simulink model "a4_jmavsim_control_smc_wordPic"  (R2023b)
settings: Solver=FixedStepAuto  StartTime=0.0  StopTime=inf  FixedStep=0.01  RelTol=1e-3  EnableMultiTasking=on
undefined symbols (not defined in the file): dev, Main, pwm_output0
libraries: simulink x19, px4uORBlib x3, sharedtransform x1, px4lib x1
settings Model: ExtModeTrigDuration=10  Creator=UAV2  LastModifiedBy=UAV2
settings SolverCC: PositivePriorityOrder=on
settings OptimizationCC: EnhancedBackFolding=on  PassReuseOutputArgsAs=Individual arguments  ZeroExternalMemoryAtStartup=off  ZeroInternalMemoryAtStartup=off  MaxStackSize=64  OptimizeBlockOrder=speed  DifferentSizesBufferReuse=on  EfficientTunableParamExpr=on
settings DebuggingCC: ParameterTunabilityLossMsg=error
settings HardwareCC: ProdBitPerPointer=32  ProdBitPerSizeT=32  ProdBitPerPtrDiffT=32  ProdLargestAtomicInteger=Long  ProdLargestAtomicFloat=Double  ProdWordSize=32  ProdLongLongMode=on  ProdHWDeviceType=ARM Compatible->ARM Cortex
settings SFSimCC: MATLABDynamicMemAlloc=off  SimTargetLang=C++
settings RTWCC: Description=Embedded Coder  SystemTargetFile=ert.tlc  HardwareBoard=PX4 Host Target  TemplateMakefile=ert_default_tmf  Toolchain=GNU Tools for PX4 Autopilots  PortableWordSizes=on  TargetLang=C++
settings CodeAppCC: ForceParamTrailComments=on  IgnoreCustomStorageClasses=off  OperatorAnnotations=on  SimulinkDataObjDesc=on  SFDataObjDesc=on  InsertBlockDesc=on
settings ERTTargetCC: ExtMode=on  ExtModeTransport=2  ExtModeStaticAlloc=on  ExtModeMexFile=ext_xcp  ExtModeMexArgs='127.0.0.1' 1 17725  ExtModeIntrfLevel=Level2 - Open

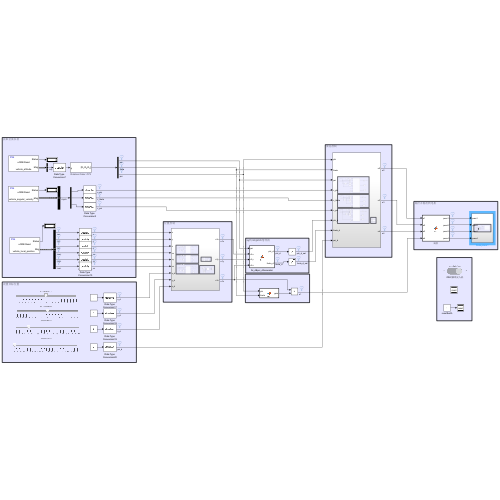
[thumbnail: Simulink's stored preview of the top-level diagram]
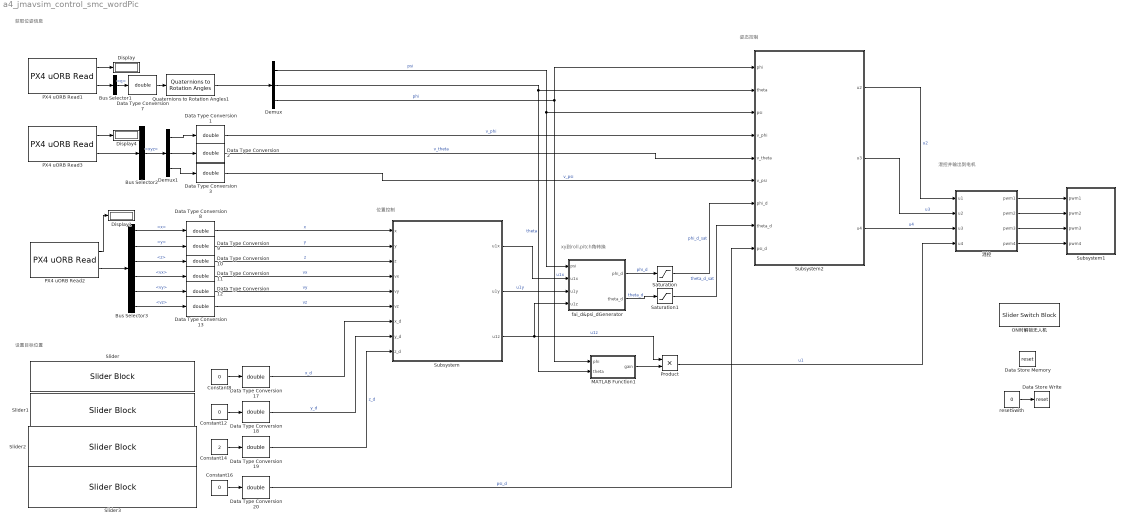
== system a4_jmavsim_control_smc_wordPic ==
  note: 混控并输出到电机
  note: xy到roll,pitch角转换
  note: 姿态控制
  note: 位置控制
  note: 设置目标位置
  note: 获取位姿信息
  Bus Selector1 : BusSelector  OutputSignals=q
  Bus Selector2 : BusSelector  OutputSignals=xyz
  Bus Selector3 : BusSelector  OutputSignals=x,y,z,vx,vy,vz
  Constant12 : Constant  Value=0
  Constant14 : Constant  Value=2
  Constant16 : Constant  Value=0
  Constant8 : Constant  Value=0
  Data Store Memory : DataStoreMemory  DataStoreName=reset  WriteAfterWriteMsg=warning  ShowAdditionalParam=off  OutDataTypeStr=boolean
  Data Store Write : DataStoreWrite  DataStoreName=reset  IndexOptions=Index vector (dialog)  Indices=1  OutputSizes=1
  Data Type Conversion{1..3,7..13,17..20} (14 alike) : DataTypeConversion  OutDataTypeStr=double  SaturateOnIntegerOverflow=off  RndMeth=Floor
  Demux : Demux  Outputs=3
  Demux1 : Demux  Outputs=3
  Display : Display
  Display1 : Display
  Display4 : Display
  MATLAB Function1 : MATLAB Function  TreatAsAtomicUnit=on
  ON时解锁无人机 : SliderSwitchBlock  Description=1时解锁无人机
      settings: Values={{'Off', 'On'}, [1 0]}
  PX4 uORB Read1 : px4uORBlib/PX4 uORB Read  uORBTopic=vehicle_attitude  selectInstance=vehicle_attitude_groundtruth  SampleTime=-1  BlockingMode=off  BlockTimeout=1e-3
  PX4 uORB Read2 : px4uORBlib/PX4 uORB Read  uORBTopic=vehicle_local_position  selectInstance=vehicle_local_position_groundtruth  SampleTime=-1  BlockingMode=off  BlockTimeout=1e-3
  PX4 uORB Read3 : px4uORBlib/PX4 uORB Read  uORBTopic=vehicle_angular_velocity  selectInstance=vehicle_angular_velocity  SampleTime=-1  BlockingMode=off  BlockTimeout=1e-3
  Product : Product
  Quaternions to Rotation Angles1 : sharedtransform/Quaternions to Rotation Angles  rotationOrder=ZYX  aMode=aMode
  Saturation : Saturate
  Saturation1 : Saturate
  Slider : SliderBlock  ScaleMin=-10  ScaleMax=10
  Slider1 : SliderBlock  ScaleMin=-10  ScaleMax=10
  Slider2 : SliderBlock  ScaleMax=10
  Slider3 : SliderBlock  ScaleMax=2
  Subsystem : Subsystem
  Subsystem1 : Subsystem
  Subsystem2 : Subsystem
  fai_d&psi_dGenerator : MATLAB Function  TreatAsAtomicUnit=on
  resetSwith : Constant  Value=0  OutDataTypeStr=boolean
  混控 : MATLAB Function  TreatAsAtomicUnit=on
  wires:
  Quaternions to Rotation Angles1/1 -> Demux/1
  PX4 uORB Read1/1 -> Display/1
  PX4 uORB Read1/2 -> Bus Selector1/1
  Bus Selector1/1 -> Data Type Conversion7/1  "<q>"
  Data Type Conversion7/1 -> Quaternions to Rotation Angles1/1
  resetSwith/1 -> Data Store Write/1
  PX4 uORB Read2/2 -> Bus Selector3/1
  Bus Selector3/2 -> Data Type Conversion9/1  "<y>"
  Bus Selector3/3 -> Data Type Conversion10/1  "<z>"
  Bus Selector3/4 -> Data Type Conversion11/1  "<vx>"
  Bus Selector3/5 -> Data Type Conversion12/1  "<vy>"
  Bus Selector3/6 -> Data Type Conversion13/1  "<vz>"
  Bus Selector3/1 -> Data Type Conversion8/1  "<x>"
  PX4 uORB Read2/1 -> Display1/1
  Subsystem/2(u1y) -> fai_d&psi_dGenerator/3(u1y)  "u1y"
  混控/1(pwm1) -> Subsystem1/1(pwm1)
  混控/2(pwm2) -> Subsystem1/2(pwm2)
  混控/3(pwm3) -> Subsystem1/3(pwm3)
  混控/4(pwm4) -> Subsystem1/4(pwm4)
  Demux/1 -> fai_d&psi_dGenerator/1(psi), Subsystem2/3(psi)  "psi"
  Demux/2 -> MATLAB Function1/2(theta), Subsystem2/2(theta)  "theta"
  Demux/3 -> MATLAB Function1/1(phi), Subsystem2/1(phi)  "phi"
  Constant16/1 -> Data Type Conversion20/1
  Data Type Conversion20/1 -> Subsystem2/9(psi_d)  "psi_d"
  fai_d&psi_dGenerator/1(phi_d) -> Saturation/1  "phi_d"
  fai_d&psi_dGenerator/2(theta_d) -> Saturation1/1  "theta_d"
  Subsystem/3(u1z) -> fai_d&psi_dGenerator/4(u1z), Product/1  "u1z"
  Saturation1/1 -> Subsystem2/8(theta_d)  "theta_d_sat"
  Data Type Conversion8/1 -> Subsystem/1(x)  "x"
  Data Type Conversion9/1 -> Subsystem/2(y)  "y"
  Data Type Conversion10/1 -> Subsystem/3(z)  "z"
  Data Type Conversion12/1 -> Subsystem/5(vy)  "vy"
  Data Type Conversion13/1 -> Subsystem/6(vz)  "vz"
  Data Type Conversion17/1 -> Subsystem/7(x_d)  "x_d"
  Data Type Conversion18/1 -> Subsystem/8(y_d)  "y_d"
  Data Type Conversion19/1 -> Subsystem/9(z_d)  "z_d"
  Data Type Conversion11/1 -> Subsystem/4(vx)  "vx"
  Subsystem/1(u1x) -> fai_d&psi_dGenerator/2(u1x)  "u1x"
  PX4 uORB Read3/2 -> Bus Selector2/1
  PX4 uORB Read3/1 -> Display4/1
  Data Type Conversion1/1 -> Subsystem2/4(v_phi)  "v_phi"
  Data Type Conversion2/1 -> Subsystem2/5(v_theta)  "v_theta"
  Data Type Conversion3/1 -> Subsystem2/6(v_psi)  "v_psi"
  Bus Selector2/1 -> Demux1/1  "<xyz>"
  Demux1/1 -> Data Type Conversion1/1
  Demux1/2 -> Data Type Conversion2/1
  Demux1/3 -> Data Type Conversion3/1
  Saturation/1 -> Subsystem2/7(phi_d)  "phi_d_sat"
  Subsystem2/3(u4) -> 混控/3(u3)  "u4"
  Subsystem2/1(u2) -> 混控/1(u1)  "u2"
  Subsystem2/2(u3) -> 混控/2(u2)  "u3"
  MATLAB Function1/1(gain) -> Product/2
  Product/1 -> 混控/4(u4)  "u1"
  Constant14/1 -> Data Type Conversion19/1
  Constant12/1 -> Data Type Conversion18/1
  Constant8/1 -> Data Type Conversion17/1

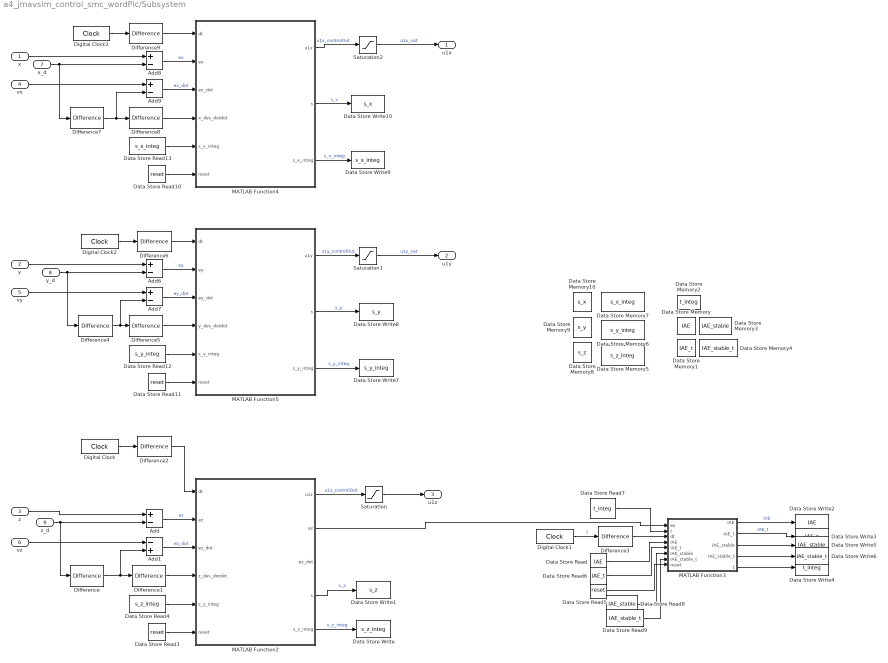
== system a4_jmavsim_control_smc_wordPic/Subsystem ==
  x : Inport
  y : Inport  Port=2
  z : Inport  Port=3
  vx : Inport  Port=4
  vy : Inport  Port=5
  vz : Inport  Port=6
  x_d : Inport  Port=7
  y_d : Inport  Port=8
  z_d : Inport  Port=9
  Add{,6..9} (5 alike) : Sum  Inputs=+-
  Add1 : Sum  Inputs=-+
  Data Store Memory : DataStoreMemory  DataStoreName=IAE  WriteAfterWriteMsg=warning  ShowAdditionalParam=off
  Data Store Memory1 : DataStoreMemory  DataStoreName=IAE_t  WriteAfterWriteMsg=warning  ShowAdditionalParam=off
  Data Store Memory10 : DataStoreMemory  DataStoreName=s_x  WriteAfterWriteMsg=warning  ShowAdditionalParam=off  OutDataTypeStr=double
  Data Store Memory2 : DataStoreMemory  DataStoreName=t_integ  WriteAfterWriteMsg=warning  ShowAdditionalParam=off
  Data Store Memory3 : DataStoreMemory  DataStoreName=IAE_stable  WriteAfterWriteMsg=warning  ShowAdditionalParam=off
  Data Store Memory4 : DataStoreMemory  DataStoreName=IAE_stable_t  WriteAfterWriteMsg=warning  ShowAdditionalParam=off
  Data Store Memory5 : DataStoreMemory  DataStoreName=s_z_integ  WriteAfterWriteMsg=warning  ShowAdditionalParam=off  OutDataTypeStr=double
  Data Store Memory6 : DataStoreMemory  DataStoreName=s_y_integ  WriteAfterWriteMsg=warning  ShowAdditionalParam=off  OutDataTypeStr=double
  Data Store Memory7 : DataStoreMemory  DataStoreName=s_x_integ  WriteAfterWriteMsg=warning  ShowAdditionalParam=off  OutDataTypeStr=double
  Data Store Memory8 : DataStoreMemory  DataStoreName=s_z  WriteAfterWriteMsg=warning  ShowAdditionalParam=off  OutDataTypeStr=double
  Data Store Memory9 : DataStoreMemory  DataStoreName=s_y  WriteAfterWriteMsg=warning  ShowAdditionalParam=off  OutDataTypeStr=double
  Data Store Read : DataStoreRead  DataStoreName=IAE  IndexOptions=Index vector (dialog)  Indices=1  OutputSizes=1
  Data Store Read{3,5,10..11} (4 alike) : DataStoreRead  DataStoreName=reset  IndexOptions=Index vector (dialog)  Indices=1  OutputSizes=1
  Data Store Read12 : DataStoreRead  DataStoreName=s_y_integ  IndexOptions=Index vector (dialog)  Indices=1  OutputSizes=1
  Data Store Read13 : DataStoreRead  DataStoreName=s_x_integ  IndexOptions=Index vector (dialog)  Indices=1  OutputSizes=1
  Data Store Read4 : DataStoreRead  DataStoreName=s_z_integ  IndexOptions=Index vector (dialog)  Indices=1  OutputSizes=1
  Data Store Read6 : DataStoreRead  DataStoreName=IAE_t  IndexOptions=Index vector (dialog)  Indices=1  OutputSizes=1
  Data Store Read7 : DataStoreRead  DataStoreName=t_integ  IndexOptions=Index vector (dialog)  Indices=1  OutputSizes=1
  Data Store Read8 : DataStoreRead  DataStoreName=IAE_stable  IndexOptions=Index vector (dialog)  Indices=1  OutputSizes=1
  Data Store Read9 : DataStoreRead  DataStoreName=IAE_stable_t  IndexOptions=Index vector (dialog)  Indices=1  OutputSizes=1
  Data Store Write : DataStoreWrite  DataStoreName=s_z_integ  IndexOptions=Index vector (dialog)  Indices=1  OutputSizes=1
  Data Store Write1 : DataStoreWrite  DataStoreName=s_z  IndexOptions=Index vector (dialog)  Indices=1  OutputSizes=1
  Data Store Write10 : DataStoreWrite  DataStoreName=s_x  IndexOptions=Index vector (dialog)  Indices=1  OutputSizes=1
  Data Store Write2 : DataStoreWrite  DataStoreName=IAE  IndexOptions=Index vector (dialog)  Indices=1  OutputSizes=1
  Data Store Write3 : DataStoreWrite  DataStoreName=IAE_t  IndexOptions=Index vector (dialog)  Indices=1  OutputSizes=1
  Data Store Write4 : DataStoreWrite  DataStoreName=t_integ  IndexOptions=Index vector (dialog)  Indices=1  OutputSizes=1
  Data Store Write5 : DataStoreWrite  DataStoreName=IAE_stable  IndexOptions=Index vector (dialog)  Indices=1  OutputSizes=1
  Data Store Write6 : DataStoreWrite  DataStoreName=IAE_stable_t  IndexOptions=Index vector (dialog)  Indices=1  OutputSizes=1
  Data Store Write7 : DataStoreWrite  DataStoreName=s_y_integ  IndexOptions=Index vector (dialog)  Indices=1  OutputSizes=1
  Data Store Write8 : DataStoreWrite  DataStoreName=s_y  IndexOptions=Index vector (dialog)  Indices=1  OutputSizes=1
  Data Store Write9 : DataStoreWrite  DataStoreName=s_x_integ  IndexOptions=Index vector (dialog)  Indices=1  OutputSizes=1
  Difference{,1..9} (10 alike) : simulink/Discrete/Difference  ICPrevInput=0.0  OutMin=[]  OutMax=[]  OutDataType=fixdt(1, 16)  OutScaling=2^-10  DoSatur=off
  Digital Clock{,1..3} (4 alike) : DigitalClock  SampleTime=0.01
  MATLAB Function2 : MATLAB Function  TreatAsAtomicUnit=on
  MATLAB Function3 : MATLAB Function  TreatAsAtomicUnit=on
  MATLAB Function4 : MATLAB Function  TreatAsAtomicUnit=on
  MATLAB Function5 : MATLAB Function  TreatAsAtomicUnit=on
  Saturation : Saturate  UpperLimit=1  LowerLimit=0
  Saturation1 : Saturate
  Saturation2 : Saturate  UpperLimit=1  LowerLimit=-1
  u1x : Outport
  u1y : Outport  Port=2
  u1z : Outport  Port=3
  wires:
  MATLAB Function2/1(u1z) -> Saturation/1  "u1z_controlOut"
  Difference/1 -> Add1/2, Difference1/1
  Difference1/1 -> MATLAB Function2/4(z_des_dotdot)
  Data Store Read3/1 -> MATLAB Function2/6(reset)
  Data Store Read4/1 -> MATLAB Function2/5("s_z_integ ")
  Digital Clock/1 -> Difference2/1
  Difference2/1 -> MATLAB Function2/1(dt)
  MATLAB Function2/4(s) -> Data Store Write1/1  "s_z"
  MATLAB Function2/5(s_z_integ) -> Data Store Write/1  "s_z_integ"
  MATLAB Function2/2(ez) -> MATLAB Function3/1(ez)
  Saturation/1 -> u1z/1
  Add/1 -> MATLAB Function2/2("ez ")  "ez"
  z_d/1 -> Add/2, Difference/1
  vz/1 -> Add1/1
  Add1/1 -> MATLAB Function2/3("ez_dot ")  "ez_dot"
  Data Store Read5/1 -> MATLAB Function3/8(reset)
  Difference3/1 -> MATLAB Function3/3(dt)
  MATLAB Function3/1(IAE) -> Data Store Write2/1  "IAE"
  MATLAB Function3/2(IAE_t) -> Data Store Write3/1  "IAE_t"
  Digital Clock1/1 -> Difference3/1  "t"
  Data Store Read/1 -> MATLAB Function3/4("IAE ")
  Data Store Read6/1 -> MATLAB Function3/5("IAE_t ")
  Data Store Read7/1 -> MATLAB Function3/2("t ")
  MATLAB Function3/5(t) -> Data Store Write4/1
  MATLAB Function3/3(IAE_stable) -> Data Store Write5/1
  MATLAB Function3/4(IAE_stable_t) -> Data Store Write6/1
  Data Store Read8/1 -> MATLAB Function3/6("IAE_stable ")
  Data Store Read9/1 -> MATLAB Function3/7("IAE_stable_t ")
  Add7/1 -> MATLAB Function5/3(ey_dot)  "ey_dot"
  Difference4/1 -> Add7/2, Difference5/1
  Data Store Read12/1 -> MATLAB Function5/5("s_y_integ ")
  MATLAB Function5/1(u1y) -> Saturation1/1  "u1y_controlOut"
  Data Store Read11/1 -> MATLAB Function5/6(reset)
  MATLAB Function5/3(s_y_integ) -> Data Store Write7/1  "s_y_integ"
  Difference5/1 -> MATLAB Function5/4(y_des_dotdot)
  Digital Clock2/1 -> Difference6/1
  vy/1 -> Add7/1
  Add6/1 -> MATLAB Function5/2(ey)  "ey"
  Saturation1/1 -> u1y/1  "u1y_sat"
  Difference6/1 -> MATLAB Function5/1(dt)
  y/1 -> Add6/1
  MATLAB Function5/2(s) -> Data Store Write8/1  "s_y"
  Difference8/1 -> MATLAB Function4/4(x_des_dotdot)
  Data Store Read10/1 -> MATLAB Function4/6(reset)
  MATLAB Function4/1(u1x) -> Saturation2/1  "u1x_controlOut"
  Data Store Read13/1 -> MATLAB Function4/5("s_x_integ ")
  Difference7/1 -> Add9/2, Difference8/1
  Add9/1 -> MATLAB Function4/3(ex_dot)  "ex_dot"
  Saturation2/1 -> u1x/1  "u1x_sat"
  MATLAB Function4/3(s_x_integ) -> Data Store Write9/1  "s_x_integ"
  Digital Clock3/1 -> Difference9/1
  Add8/1 -> MATLAB Function4/2(ex)  "ex"
  Difference9/1 -> MATLAB Function4/1(dt)
  MATLAB Function4/2(s) -> Data Store Write10/1  "s_x"
  z/1 -> Add/1
  x/1 -> Add8/1
  vx/1 -> Add9/1
  x_d/1 -> Add8/2, Difference7/1
  y_d/1 -> Add6/2, Difference4/1

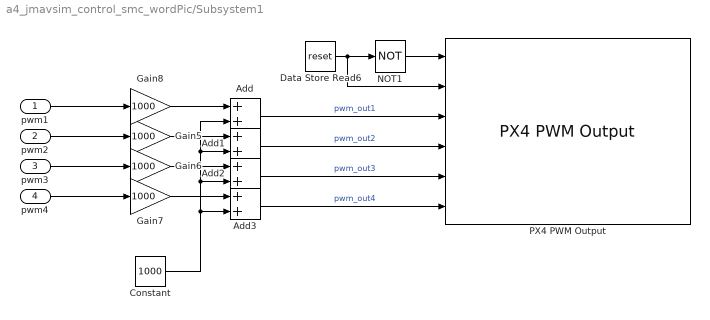
== system a4_jmavsim_control_smc_wordPic/Subsystem1 ==
  pwm1 : Inport
  pwm2 : Inport  Port=2
  pwm3 : Inport  Port=3
  pwm4 : Inport  Port=4
  Add{,1..3} (4 alike) : Sum  OutDataTypeStr=uint16
  Constant : Constant  Value=1000
  Data Store Read6 : DataStoreRead  DataStoreName=reset  IndexOptions=Index vector (dialog)  Indices=1  OutputSizes=1
  Gain{5..8} (4 alike) : Gain  Gain=1000  OutDataTypeStr=uint16
  NOT1 : Logic  Operator=NOT  IconShape=distinctive  AllPortsSameDT=off  OutDataTypeStr=boolean
  PX4 PWM Output : px4lib/PX4 PWM Output  pwmDevice=Main (/dev/pwm_output0)  pwmChannel1_=on  pwmChannel2_=on  pwmChannel3_=on  pwmChannel4_=on  pwmChannel5_=off  pwmChannel6_=off  pwmChannel7_=off  pwmChannel8_=off  forceTerminateFailsafe=off  outputErrorStatus=off
  wires:
  NOT1/1 -> PX4 PWM Output/1
  Add3/1 -> PX4 PWM Output/6  "pwm_out4"
  Data Store Read6/1 -> PX4 PWM Output/2, NOT1/1
  Add/1 -> PX4 PWM Output/3  "pwm_out1"
  Add1/1 -> PX4 PWM Output/4  "pwm_out2"
  pwm3/1 -> Gain6/1
  pwm1/1 -> Gain8/1
  pwm2/1 -> Gain5/1
  pwm4/1 -> Gain7/1
  Add2/1 -> PX4 PWM Output/5  "pwm_out3"
  Gain8/1 -> Add/1
  Constant/1 -> Add3/2, Add2/2, Add1/2, Add/2
  Gain5/1 -> Add1/1
  Gain7/1 -> Add3/1
  Gain6/1 -> Add2/1

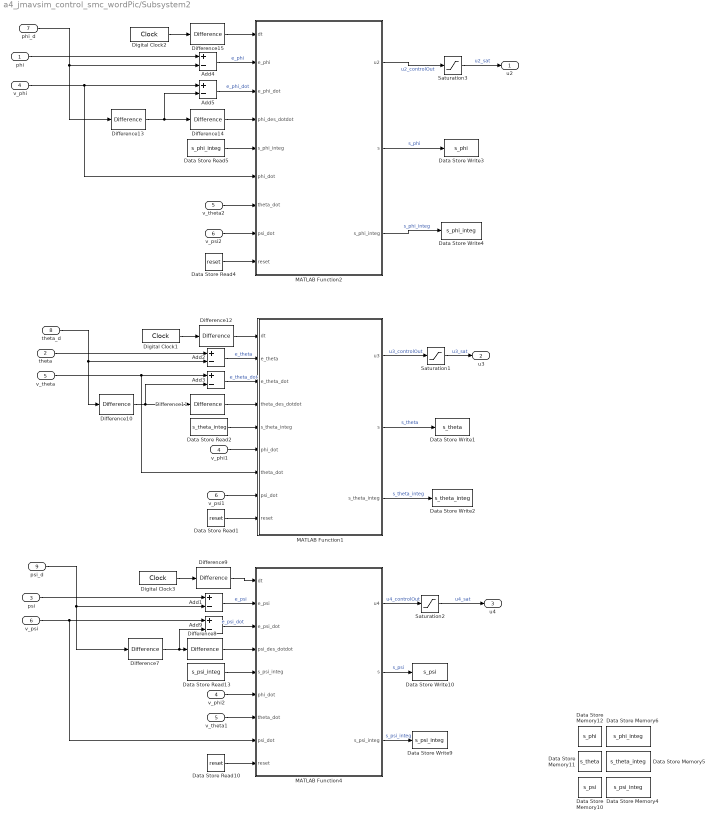
== system a4_jmavsim_control_smc_wordPic/Subsystem2 ==
  phi : Inport
  theta : Inport  Port=2
  psi : Inport  Port=3
  v_phi : Inport  Port=4
  v_theta : Inport  Port=5
  v_psi : Inport  Port=6
  phi_d : Inport  Port=7
  theta_d : Inport  Port=8
  psi_d : Inport  Port=9
  Add{1..5,9} (6 alike) : Sum  Inputs=+-
  Data Store Memory10 : DataStoreMemory  DataStoreName=s_psi  WriteAfterWriteMsg=warning  ShowAdditionalParam=off  OutDataTypeStr=double
  Data Store Memory11 : DataStoreMemory  DataStoreName=s_theta  WriteAfterWriteMsg=warning  ShowAdditionalParam=off  OutDataTypeStr=double
  Data Store Memory12 : DataStoreMemory  DataStoreName=s_phi  WriteAfterWriteMsg=warning  ShowAdditionalParam=off  OutDataTypeStr=double
  Data Store Memory4 : DataStoreMemory  DataStoreName=s_psi_integ  WriteAfterWriteMsg=warning  ShowAdditionalParam=off  OutDataTypeStr=double
  Data Store Memory5 : DataStoreMemory  DataStoreName=s_theta_integ  WriteAfterWriteMsg=warning  ShowAdditionalParam=off  OutDataTypeStr=double
  Data Store Memory6 : DataStoreMemory  DataStoreName=s_phi_integ  WriteAfterWriteMsg=warning  ShowAdditionalParam=off  OutDataTypeStr=double
  Data Store Read1 : DataStoreRead  DataStoreName=reset  IndexOptions=Index vector (dialog)  Indices=1  OutputSizes=1
  Data Store Read10 : DataStoreRead  DataStoreName=reset  IndexOptions=Index vector (dialog)  Indices=1  OutputSizes=1
  Data Store Read13 : DataStoreRead  DataStoreName=s_psi_integ  IndexOptions=Index vector (dialog)  Indices=1  OutputSizes=1
  Data Store Read2 : DataStoreRead  DataStoreName=s_theta_integ  IndexOptions=Index vector (dialog)  Indices=1  OutputSizes=1
  Data Store Read4 : DataStoreRead  DataStoreName=reset  IndexOptions=Index vector (dialog)  Indices=1  OutputSizes=1
  Data Store Read5 : DataStoreRead  DataStoreName=s_phi_integ  IndexOptions=Index vector (dialog)  Indices=1  OutputSizes=1
  Data Store Write1 : DataStoreWrite  DataStoreName=s_theta  IndexOptions=Index vector (dialog)  Indices=1  OutputSizes=1
  Data Store Write10 : DataStoreWrite  DataStoreName=s_psi  IndexOptions=Index vector (dialog)  Indices=1  OutputSizes=1
  Data Store Write2 : DataStoreWrite  DataStoreName=s_theta_integ  IndexOptions=Index vector (dialog)  Indices=1  OutputSizes=1
  Data Store Write3 : DataStoreWrite  DataStoreName=s_phi  IndexOptions=Index vector (dialog)  Indices=1  OutputSizes=1
  Data Store Write4 : DataStoreWrite  DataStoreName=s_phi_integ  IndexOptions=Index vector (dialog)  Indices=1  OutputSizes=1
  Data Store Write9 : DataStoreWrite  DataStoreName=s_psi_integ  IndexOptions=Index vector (dialog)  Indices=1  OutputSizes=1
  Difference{7..15} (9 alike) : simulink/Discrete/Difference  ICPrevInput=0.0  OutMin=[]  OutMax=[]  OutDataType=fixdt(1, 16)  OutScaling=2^-10  DoSatur=off
  Digital Clock1 : DigitalClock  SampleTime=0.01
  Digital Clock2 : DigitalClock  SampleTime=0.01
  Digital Clock3 : DigitalClock  SampleTime=0.01
  MATLAB Function1 : MATLAB Function  TreatAsAtomicUnit=on
  MATLAB Function2 : MATLAB Function  TreatAsAtomicUnit=on
  MATLAB Function4 : MATLAB Function  TreatAsAtomicUnit=on
  Saturation1 : Saturate  UpperLimit=0.1  LowerLimit=-0.1
  Saturation2 : Saturate  UpperLimit=0.2  LowerLimit=-0.2
  Saturation3 : Saturate  UpperLimit=0.1  LowerLimit=-0.1
  v_phi1 : InportShadow  Port=4
  v_phi2 : InportShadow  Port=4
  v_psi1 : InportShadow  Port=6
  v_psi2 : InportShadow  Port=6
  v_theta1 : InportShadow  Port=5
  v_theta2 : InportShadow  Port=5
  u2 : Outport
  u3 : Outport  Port=2
  u4 : Outport  Port=3
  wires:
  Data Store Read10/1 -> MATLAB Function4/9(reset)
  Data Store Read13/1 -> MATLAB Function4/5("s_psi_integ ")
  MATLAB Function4/3(s_psi_integ) -> Data Store Write9/1  "s_psi_integ"
  Saturation2/1 -> u4/1  "u4_sat"
  Add9/1 -> MATLAB Function4/3(e_psi_dot)  "e_psi_dot"
  Difference7/1 -> Add9/2, Difference8/1
  Difference8/1 -> MATLAB Function4/4(psi_des_dotdot)
  Difference9/1 -> MATLAB Function4/1(dt)
  MATLAB Function4/2(s) -> Data Store Write10/1  "s_psi"
  MATLAB Function4/1(u4) -> Saturation2/1  "u4_controlOut"
  Digital Clock3/1 -> Difference9/1
  psi/1 -> Add1/1
  Add1/1 -> MATLAB Function4/2(e_psi)  "e_psi"
  Difference12/1 -> MATLAB Function1/1(dt)
  Digital Clock1/1 -> Difference12/1
  Difference11/1 -> MATLAB Function1/4(theta_des_dotdot)
  MATLAB Function1/1(u3) -> Saturation1/1  "u3_controlOut"
  Data Store Read2/1 -> MATLAB Function1/5("s_theta_integ ")
  MATLAB Function1/2(s) -> Data Store Write1/1  "s_theta"
  Difference10/1 -> Add3/2, Difference11/1
  Data Store Read1/1 -> MATLAB Function1/9(reset)
  Add2/1 -> MATLAB Function1/2(e_theta)  "e_theta"
  Add3/1 -> MATLAB Function1/3(e_theta_dot)  "e_theta_dot"
  MATLAB Function1/3(s_theta_integ) -> Data Store Write2/1  "s_theta_integ"
  theta/1 -> Add2/1
  Saturation3/1 -> u2/1  "u2_sat"
  phi/1 -> Add4/1
  Difference13/1 -> Add5/2, Difference14/1
  Data Store Read4/1 -> MATLAB Function2/9(reset)
  MATLAB Function2/1(u2) -> Saturation3/1  "u2_controlOut"
  Data Store Read5/1 -> MATLAB Function2/5("s_phi_integ ")
  Difference14/1 -> MATLAB Function2/4(phi_des_dotdot)
  Digital Clock2/1 -> Difference15/1
  Difference15/1 -> MATLAB Function2/1(dt)
  Add5/1 -> MATLAB Function2/3(e_phi_dot)  "e_phi_dot"
  MATLAB Function2/2(s) -> Data Store Write3/1  "s_phi"
  Add4/1 -> MATLAB Function2/2(e_phi)  "e_phi"
  MATLAB Function2/3(s_phi_integ) -> Data Store Write4/1  "s_phi_integ"
  v_phi/1 -> MATLAB Function2/6(phi_dot), Add5/1
  v_theta/1 -> Add3/1, MATLAB Function1/7(theta_dot)
  v_psi/1 -> Add9/1, MATLAB Function4/8(psi_dot)
  v_phi1/1 -> MATLAB Function1/6(phi_dot)
  v_theta2/1 -> MATLAB Function2/7(theta_dot)
  v_psi2/1 -> MATLAB Function2/8(psi_dot)
  v_psi1/1 -> MATLAB Function1/8(psi_dot)
  v_phi2/1 -> MATLAB Function4/6(phi_dot)
  v_theta1/1 -> MATLAB Function4/7(theta_dot)
  Saturation1/1 -> u3/1  "u3_sat"
  psi_d/1 -> Difference7/1, Add1/2
  theta_d/1 -> Difference10/1, Add2/2
  phi_d/1 -> Difference13/1, Add4/2

== matlab function a4_jmavsim_control_smc_wordPic/Subsystem/MATLAB Function5 ==
  data: dt input; ey input double; u1y output double; ey_dot input double; y_des_dotdot input; s_y_integ input; reset input; s output; s_y_integ output
function [u1y, s, s_y_integ] = u1yfcn(dt, ey, ey_dot, y_des_dotdot,...
                    s_y_integ, reset)

if (reset == 1); s_y_integ = 0; end
m = 0.8; g = 9.80665; %Ix = 0.005; Iy = 0.005; Iz = 0.009; L = 0.33 / 2;
Ky = 0;

alpha = 2;beta = 1;gamma = 0.4;
mu = 0.9;r = 5/3;
K=0.1;K1 = 0.5;K2 = 0.5;

s = alpha * ey +  (beta * sign(ey_dot) * (abs(ey_dot)) ^ mu) + (gamma * sign(ey) * (abs(ey)) ^ r);
s_y_integ = s_y_integ + K2 * sign(s) * dt;

u1y = -m*(- Ky/m*ey_dot - y_des_dotdot + alpha/(beta*mu)*sign(ey_dot) * (abs(ey_dot))^(2-mu)...
    + gamma*r/(beta*mu)*(sign(ey) * (abs(ey))^(r-1))* sign(ey_dot) * (abs(ey_dot))^(2-mu) + K1*(abs(s))^(1/2)*sign(s)...
    + s_y_integ);

u1y = u1y * K;

== matlab function a4_jmavsim_control_smc_wordPic/Subsystem2/MATLAB Function4 ==
  data: dt input; e_psi input double; u4 output double; e_psi_dot input double; psi_des_dotdot input; s_psi_integ input; phi_dot input; theta_dot input; psi_dot input; reset input; s output; s_psi_integ output
function [u4, s, s_psi_integ] = u4fcn(dt, e_psi, e_psi_dot, psi_des_dotdot,...
                    s_psi_integ, phi_dot, theta_dot, psi_dot, reset)

if (reset == 1); s_psi_integ = 0; end
m = 0.8; g = 9.80665; Ix = 0.005; Iy = 0.005; Iz = 0.009; L = 0.33 / 2;
Kpsi = 0;

alpha = 2;beta = 1;gamma = 0.4;
mu = 15/17;r = 1.1;
K = 5; K1 = 2; K2 = 2;

s = alpha * e_psi +  real(beta * sign(e_psi_dot) * (abs(e_psi_dot)) ^ mu) + real(gamma * sign(e_psi) * (abs(e_psi)) ^ r);
s_psi_integ = s_psi_integ + K2 * sign(s) * dt;

u4 = -Iz*((Ix-Iy)/Iz*phi_dot*theta_dot - Kpsi/Iz*psi_dot - psi_des_dotdot + alpha/(beta*mu)*sign(e_psi_dot) * (abs(e_psi_dot))^(2-mu)...
    + gamma*r/(beta*mu)*(sign(e_psi) * (abs(e_psi))^(r-1))* sign(e_psi_dot) * (abs(e_psi_dot))^(2-mu) + K1*(abs(s))^(1/2)*sign(s)...
    + s_psi_integ);
u4 = u4 * K;

== matlab function a4_jmavsim_control_smc_wordPic/fai_d&psi_dGenerator ==
  data: psi input double; phi_d output double; u1x input double; u1y input double; u1z input double; theta_d output double
function [phi_d, theta_d] = fcn(psi, u1x, u1y, u1z)

% fai_d = atan((y_d - y)/(x_d - x));
% theta_d = atan((z_d - z)/(((x_d - x)^2 + (y_d - y)^2)^(1/2)));
phi_d = -1 * atan((u1x * sin(psi) - u1y * cos(psi)) / u1z );
theta_d = -1 * atan((u1x * cos(psi) + u1y * sin(psi)) * cos(phi_d) / u1z );

== matlab function a4_jmavsim_control_smc_wordPic/MATLAB Function1 ==
  data: phi input double; gain output double; theta input double
function gain = fcn(phi, theta)

gain = 1/(cos(phi) * cos(theta));

== matlab function a4_jmavsim_control_smc_wordPic/Subsystem2/MATLAB Function1 ==
  data: dt input; e_theta input double; u3 output double; e_theta_dot input double; theta_des_dotdot input; s_theta_integ input; phi_dot input; theta_dot input; psi_dot input; reset input; s output; s_theta_integ output
function [u3, s, s_theta_integ] = u3fcn(dt, e_theta, e_theta_dot, theta_des_dotdot,...
                    s_theta_integ, phi_dot, theta_dot, psi_dot, reset)

if (reset == 1); s_theta_integ = 0; end
m = 0.8; g = 9.80665; Ix = 0.005; Iy = 0.005; Iz = 0.009; L = 0.33 / 2;
Ktheta = 0;

alpha = 2;beta = 1;gamma = 0.4;
mu = 15/17;r = 1.1;
K1 = 5; K2 = (K1^2)/2;

s = alpha * e_theta +  (beta * sign(e_theta_dot) * (abs(e_theta_dot)) ^ mu) + (gamma * sign(e_theta) * (abs(e_theta)) ^ r);
s_theta_integ = s_theta_integ + K2 * sign(s) * dt;

u3 = -Iy*((Iz-Ix)/Iy*phi_dot*psi_dot - Ktheta/Iy*theta_dot - theta_des_dotdot + alpha/(beta*mu)*sign(e_theta_dot) * (abs(e_theta_dot))^(2-mu)...
    + gamma*r/(beta*mu)*(sign(e_theta) * (abs(e_theta))^(r-1))* sign(e_theta_dot) * (abs(e_theta_dot))^(2-mu) + K1*(abs(s))^(1/2)*sign(s)...
    + s_theta_integ);

== matlab function a4_jmavsim_control_smc_wordPic/Subsystem2/MATLAB Function2 ==
  data: dt input; e_phi input double; u2 output double; e_phi_dot input double; phi_des_dotdot input; s_phi_integ input; phi_dot input; theta_dot input; psi_dot input; reset input; s output; s_phi_integ output
function [u2, s, s_phi_integ] = u2fcn(dt, e_phi, e_phi_dot, phi_des_dotdot,...
                    s_phi_integ, phi_dot, theta_dot, psi_dot, reset)

if (reset == 1); s_phi_integ = 0; end
m = 0.8; g = 9.80665; Ix = 0.005; Iy = 0.005; Iz = 0.009; L = 0.33 / 2;
Kphi = 0;

alpha = 2;beta = 1;gamma = 0.4;
mu = 15/17;r = 1.1;
K1 = 5; K2 = (K1^2)/2;

s = alpha * e_phi +  (beta * sign(e_phi_dot) * (abs(e_phi_dot)) ^ mu) + (gamma * sign(e_phi) * (abs(e_phi)) ^ r);
s_phi_integ = s_phi_integ + K2 * sign(s) * dt;

u2 = -Ix*((Iy-Iz)/Ix*theta_dot*psi_dot - Kphi/Ix*phi_dot - phi_des_dotdot + alpha/(beta*mu)*sign(e_phi_dot) * (abs(e_phi_dot))^(2-mu)...
    + gamma*r/(beta*mu)*(sign(e_phi) * (abs(e_phi))^(r-1))* sign(e_phi_dot) * (abs(e_phi_dot))^(2-mu) + K1*(abs(s))^(1/2)*sign(s)...
    + s_phi_integ);

== matlab function a4_jmavsim_control_smc_wordPic/混控 ==
  data: u1 input double; pwm1 output double; u2 input double; u3 input double; u4 input double; pwm2 output double; pwm3 output; pwm4 output
function [pwm1,pwm2,pwm3,pwm4] = fcn(u1, u2, u3, u4)

convertMatrix = [-1/sqrt(2)     1/sqrt(2)   1 1;
                1/sqrt(2)       -1/sqrt(2)  1 1;
                1/sqrt(2)       1/sqrt(2)  -1 1;
                -1/sqrt(2)      -1/sqrt(2) -1 1];
pwm = convertMatrix * [u1; u2; u3; u4];
pwm1 = pwm(1);
pwm2 = pwm(2);
pwm3 = pwm(3);
pwm4 = pwm(4);

== matlab function a4_jmavsim_control_smc_wordPic/Subsystem/MATLAB Function2 ==
  data: dt input; ez input double; u1z output double; ez output; ez_dot output; ez_dot input double; z_des_dotdot input; s_z_integ input; reset input; s output; s_z_integ output
function [u1z, ez, ez_dot, s, s_z_integ] = u1zfcn(dt, ez, ez_dot, z_des_dotdot,...
                    s_z_integ, reset)

if (reset == 1); s_z_integ = 0; end
m = 0.8; g = 9.80665; %Ix = 0.005; Iy = 0.005; Iz = 0.009; L = 0.33 / 2;
Kz = 0;

alpha = 2;beta = 1;gamma = 0.4;
mu = 0.9;r = 5/3;
K=2;K1 = 1;K2 = 1;

s = alpha * ez +  (beta * sign(ez_dot) * (abs(ez_dot)) ^ mu) + (gamma * sign(ez) * (abs(ez)) ^ r);
s_z_integ = s_z_integ + K2 * sign(s) * dt;

u1z = -m*(-g - Kz/m*ez_dot - z_des_dotdot + alpha/(beta*mu)*sign(ez_dot) * (abs(ez_dot))^(2-mu)...
    + gamma*r/(beta*mu)*(sign(ez) * (abs(ez))^(r-1))* sign(ez_dot) * (abs(ez_dot))^(2-mu) + K1*(abs(s))^(1/2)*sign(s)...
    + s_z_integ);

u1z = u1z/(K*m*g);

== matlab function a4_jmavsim_control_smc_wordPic/Subsystem/MATLAB Function3 ==
  data: ez input double; t input; IAE output; dt input double; IAE input; IAE_t input; IAE_stable input; IAE_stable_t input; reset input; IAE_t output; IAE_stable output; IAE_stable_t output; t output
function [IAE, IAE_t, IAE_stable, IAE_stable_t, t]  = fcn(ez, t, dt, IAE, IAE_t, IAE_stable, IAE_stable_t, reset)

if (reset == 1); t = 0; IAE = 0; IAE_stable = 0; IAE_t = 0; IAE_stable_t = 0; end

t = t + dt;
if (t < 5.01); IAE = IAE + sqrt(ez^2)*dt; end

if (t > 5.00 && t < 10.01); IAE_stable = IAE_stable + sqrt(ez^2)*dt; end

if (t > 4.99 && t < 5.01); IAE_t =  IAE / t; end

if (t > 9.99 && t < 10.01); IAE_stable_t =  IAE_stable / 5; end

== matlab function a4_jmavsim_control_smc_wordPic/Subsystem/MATLAB Function4 ==
  data: dt input; ex input double; u1x output double; ex_dot input double; x_des_dotdot input; s_x_integ input; reset input; s output; s_x_integ output
function [u1x, s, s_x_integ] = u1xfcn(dt, ex, ex_dot, x_des_dotdot,...
                    s_x_integ, reset)

if (reset == 1); s_x_integ = 0; end
m = 0.8; g = 9.80665; %Ix = 0.005; Iy = 0.005; Iz = 0.009; L = 0.33 / 2;
Kx = 0;

alpha = 2;beta = 1;gamma = 0.4;
mu = 0.9;r = 5/3;
K=0.1;K1 = 0.5;K2 = 0.5;

s = alpha * ex +  (beta * sign(ex_dot) * (abs(ex_dot)) ^ mu) + (gamma * sign(ex) * (abs(ex)) ^ r);
s_x_integ = s_x_integ + K2 * sign(s) * dt;

u1x = -m*(- Kx/m*ex_dot - x_des_dotdot + alpha/(beta*mu)*sign(ex_dot) * (abs(ex_dot))^(2-mu)...
    + gamma*r/(beta*mu)*(sign(ex) * (abs(ex))^(r-1))* sign(ex_dot) * (abs(ex_dot))^(2-mu) + K1*(abs(s))^(1/2)*sign(s)...
    + s_x_integ);
u1x = u1x * K;
